simulink subsystem "QuadSensors"  (R2025a)
settings: Solver=VariableStepAuto  StartTime=0.0  StopTime=10.0  RelTol=1e-3
undefined symbols (not defined in the file or in its folder): dspblkCoreblockFVToolHelper, gcbh, gyro_filt_den, gyro_filt_num, Ts_FB
libraries: simulink x3, aerolibutil x1, sharedutil x1
settings Model: Creator=luker  LastModifiedBy=luke

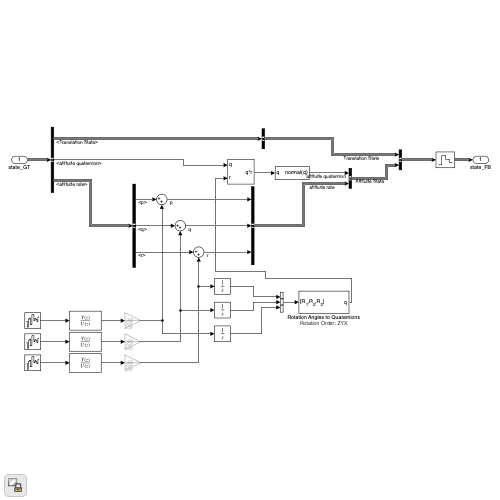
[thumbnail: Simulink's stored preview of the top-level diagram]
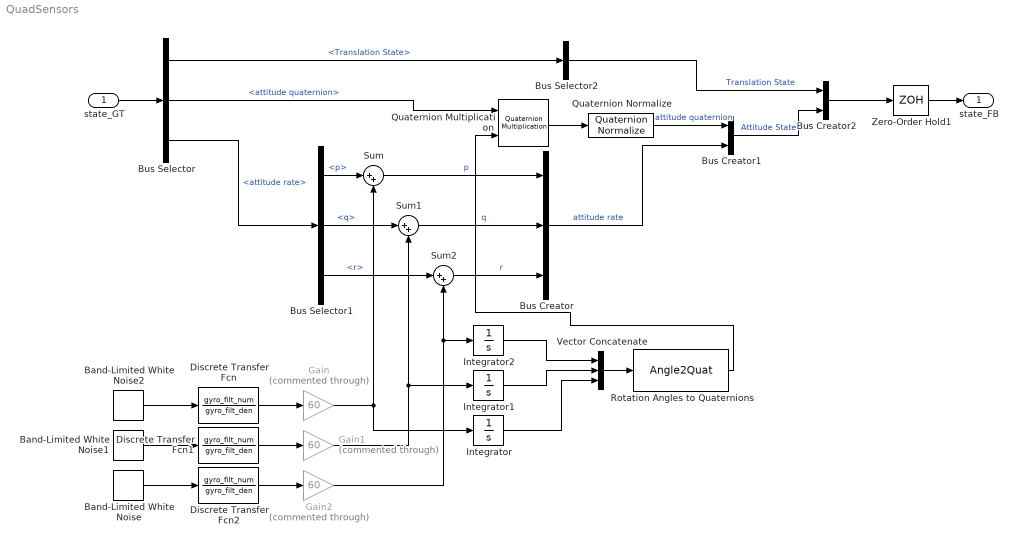
== system QuadSensors ==
  state_GT : Inport
  Band-Limited White Noise : simulink/Sources/Band-Limited White Noise  Cov=1.2e-9  Ts=0.001  seed=[23341]
  Band-Limited White Noise1 : simulink/Sources/Band-Limited White Noise  Cov=1.2e-9  Ts=0.001  seed=[23342]
  Band-Limited White Noise2 : simulink/Sources/Band-Limited White Noise  Cov=1e-9  Ts=1/1000  seed=[233413]
  Bus Creator : BusCreator  Inputs=3
  Bus Creator1 : BusCreator  Inputs=2
  Bus Creator2 : BusCreator  Inputs=2
  Bus Selector : BusSelector  OutputSignals=Translation State,Attitude State.attitude quaternion,Attitude State.attitude rate
  Bus Selector1 : BusSelector  OutputSignals=p,q,r
  Bus Selector2 : BusSelector  OutputSignals=position,velocity  OutputAsBus=on
  Discrete Transfer Fcn : DiscreteTransferFcn  LoadFcn=dspblkCoreblockFVToolHelper(gcbh,'load');  Numerator=gyro_filt_num  Denominator=gyro_filt_den
      settings: CopyFcn=dspblkCoreblockFVToolHelper(gcbh,'copy');  DeleteFcn=dspblkCoreblockFVToolHelper(gcbh,'close');  ModelCloseFcn=dspblkCoreblockFVToolHelper(gcbh,'close');  PreSaveFcn=dspblkCoreblockFVToolHelper(gcbh,'presave');  PostSaveFcn=dspblkCoreblockFVToolHelper(gcbh,'postsave');  CloseFcn=dspblkCoreblockFVToolHelper(gcbh,'close');
  Discrete Transfer Fcn1 : DiscreteTransferFcn  LoadFcn=dspblkCoreblockFVToolHelper(gcbh,'load');  Numerator=gyro_filt_num  Denominator=gyro_filt_den
      settings: CopyFcn=dspblkCoreblockFVToolHelper(gcbh,'copy');  DeleteFcn=dspblkCoreblockFVToolHelper(gcbh,'close');  ModelCloseFcn=dspblkCoreblockFVToolHelper(gcbh,'close');  PreSaveFcn=dspblkCoreblockFVToolHelper(gcbh,'presave');  PostSaveFcn=dspblkCoreblockFVToolHelper(gcbh,'postsave');  CloseFcn=dspblkCoreblockFVToolHelper(gcbh,'close');
  Discrete Transfer Fcn2 : DiscreteTransferFcn  LoadFcn=dspblkCoreblockFVToolHelper(gcbh,'load');  Numerator=gyro_filt_num  Denominator=gyro_filt_den
      settings: CopyFcn=dspblkCoreblockFVToolHelper(gcbh,'copy');  DeleteFcn=dspblkCoreblockFVToolHelper(gcbh,'close');  ModelCloseFcn=dspblkCoreblockFVToolHelper(gcbh,'close');  PreSaveFcn=dspblkCoreblockFVToolHelper(gcbh,'presave');  PostSaveFcn=dspblkCoreblockFVToolHelper(gcbh,'postsave');  CloseFcn=dspblkCoreblockFVToolHelper(gcbh,'close');
  Gain : Gain  Commented=through  Gain=60
  Gain1 : Gain  Commented=through  Gain=60
  Gain2 : Gain  Commented=through  Gain=60
  Integrator : Integrator
  Integrator1 : Integrator
  Integrator2 : Integrator
  Quaternion Multiplication : aerolibutil/Quaternion Multiplication
  Quaternion Normalize : sharedutil/Quaternion Normalize  aMode=aMode
  Rotation Angles to Quaternions : Angle2Quat
      settings: AttributesFormatString=Rotation Order: %<rotationOrder>
  Sum : Sum  Inputs=|++
  Sum1 : Sum  Inputs=|++
  Sum2 : Sum  Inputs=|++
  Vector Concatenate : Concatenate  NumInputs=3
  Zero-Order Hold1 : ZeroOrderHold  SampleTime=Ts_FB
  state_FB : Outport
  wires:
  state_GT/1 -> Bus Selector/1
  Bus Selector/3 -> Bus Selector1/1  "<attitude rate>"
  Bus Selector1/1 -> Sum/1  "<p>"
  Bus Selector1/2 -> Sum1/1  "<q>"
  Bus Selector1/3 -> Sum2/1  "<r>"
  Sum/1 -> Bus Creator/1  "p"
  Sum1/1 -> Bus Creator/2  "q"
  Sum2/1 -> Bus Creator/3  "r"
  Bus Creator/1 -> Bus Creator1/2  "attitude rate"
  Bus Creator2/1 -> Zero-Order Hold1/1
  Bus Creator1/1 -> Bus Creator2/2  "Attitude State"
  Band-Limited White Noise1/1 -> Discrete Transfer Fcn1/1
  Band-Limited White Noise/1 -> Discrete Transfer Fcn2/1
  Band-Limited White Noise2/1 -> Discrete Transfer Fcn/1
  Discrete Transfer Fcn/1 -> Gain/1
  Discrete Transfer Fcn1/1 -> Gain1/1
  Discrete Transfer Fcn2/1 -> Gain2/1
  Bus Selector/1 -> Bus Selector2/1  "<Translation State>"
  Bus Selector2/1 -> Bus Creator2/1  "Translation State"
  Zero-Order Hold1/1 -> state_FB/1
  Bus Selector/2 -> Quaternion Multiplication/1  "<attitude quaternion>"
  Gain/1 -> Integrator/1, Sum/2
  Gain1/1 -> Sum1/2, Integrator1/1
  Gain2/1 -> Integrator2/1, Sum2/2
  Quaternion Normalize/1 -> Bus Creator1/1  "attitude quaternion"
  Vector Concatenate/1 -> Rotation Angles to Quaternions/1
  Integrator2/1 -> Vector Concatenate/1
  Integrator1/1 -> Vector Concatenate/2
  Integrator/1 -> Vector Concatenate/3
  Rotation Angles to Quaternions/1 -> Quaternion Multiplication/2
  Quaternion Multiplication/1 -> Quaternion Normalize/1
